simulink model "Correlation_Ex1"  (R2024a)
settings: Solver=VariableStepAuto  StartTime=0.0  StopTime=1024  RelTol=1e-3
InitFcn:
  | F_Length = 16;
  | G_Length = 16;
undefined symbols (not defined in the file): S, vsva2197, xcvc1902
libraries: dspstat3 x1, aieDSP x1, aieUtilities x1, vmcUtilities x1
settings Model: Creator=sdegala  LastModifiedBy=sdegala

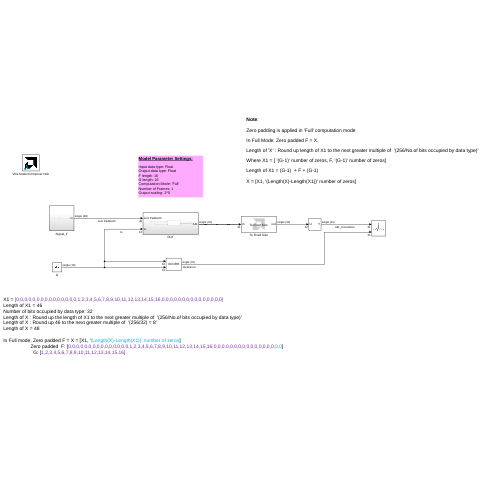
[thumbnail: Simulink's stored preview of the top-level diagram]
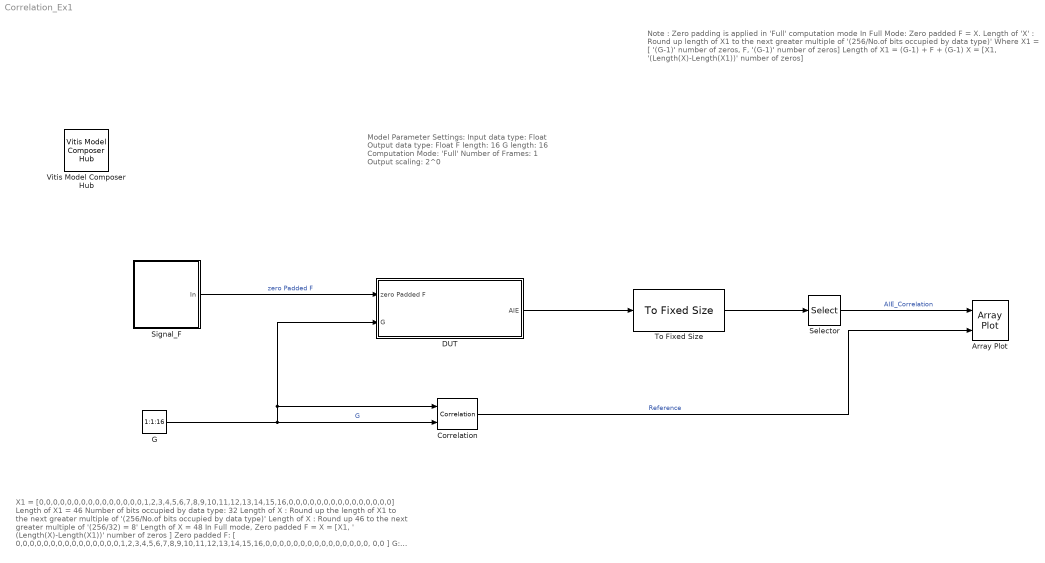
== system Correlation_Ex1 ==
  note: X1 = [0,0,0,0,0,0,0,0,0,0,0,0,0,0,0,1,2,3,4,5,6,7,8,9,10,11,12,13,14,15,16,0,0,0,0,0,0,0,0,0,0,0,0,0,0,0]
      | Length of X1 = 46
      | Number of bits occupied by data type: 32
      | Length of X : Round up the length of X1 to the next greater multiple of '(256/No.of bits occupied by data type)'
      | Length of X : Round up 46 to the next greater multiple of '(256/32) = 8'
      | Length of X = 48
      |
      | In Full mode, Zero padded F = X = [X1, ' (Length(X)-Length(X1))' number of zeros ]
      | Zero padded F: [ 0,0,0,0,0,0,0,0,0,0,0,0,0,0,0,1,2,3,4,5,6,7,8,9,10,11,12,13,14,15,16,0,0,0,0,0,0,0,0,0,0,0,0,0,0,0, 0,0 ]
      | G: [ 1,2,3,4,5,6,7,8,9,10,11,12,13,14,15,16]
  note: Note :
      |
      | Zero padding is applied in 'Full' computation mode
      |
      | In Full Mode: Zero padded F = X.
      |
      | Length of 'X' : Round up length of X1 to the next greater multiple of '(256/No.of bits occupied by data type)'
      |
      | Where X1 = [ '(G-1)' number of zeros, F, '(G-1)' number of zeros]
      |
      | Length of X1 = (G-1) + F + (G-1)
      |
      | X = [X1, '(Length(X)-Length(X1))' number of zeros]
  note: Model Parameter Settings:
      |
      | Input data type: Float
      | Output data type: Float
      | F length: 16
      | G length: 16
      | Computation Mode: 'Full'
      | Number of Frames: 1
      | Output scaling: 2^0
  Array Plot : ArrayPlot  NumInputPorts=2  WindowPosition=[663.000000,396.000000,800.000000,500.000000,]  Visible=on  ScopeFrameLocation=window  YLimits=[-169 1681]  ShowLegend=on
  Correlation : dspstat3/Correlation  domain=Time  roundingMode=Floor  overflowMode=off  outputDataTypeStr=Inherit: Same as accumulator  outputMin=[]  outputMax=[]  outputLastDataTypeStr=Inherit: Same as accumulator
  DUT : Subsystem
  G : Constant  Value=1:1:16  OutDataTypeStr=single  SampleTime=1
  Selector : Selector  InputPortWidth=32  IndexOptions=Index vector (dialog)  Indices=1:1:F_Length+G_Length-1  OutputSizes=1
  Signal_F : Subsystem
  To Fixed Size : aieUtilities/To Fixed Size  Mode=Stop simulation when input variable-size signal is not full  OutputSize=Inherit: Same as input  CopyMethod=Buffer samples to form output  HasStatusOutput=on
  Vitis Model Composer Hub : vmcUtilities/Vitis Model Composer Hub  Tag=genX  CodeGeneration=off  StartColumn=1  NumberOfColumns=1  TargetDirectory=./code  exportDesign=off  analyzeDesign=off  validateDesignOnHw=off  ExportType=AI Engines  IpVendor=xilinx.com  IpLibrary=hls  IpVersion=1.0  IpHWLanguage=Verilog  AieCompilerOptions={}  AieSimulatorOptions={}  CreateTestbench=off  TestbenchStackSize=10  RunRtlSim=off  RunCSim=off  RunAieSim=off  AieSimTimeout=50000  RunAieSimProfiling=off  LaunchVitisAnalyzer=off  PlotOutput=off  RunX86Sim=off  X86SimTimeout=10  GenHwImage=off  GenLibadfXo=off  GenHwValidationCode=off  PlatformType=Not Specified  HwSystemType=Baremetal  HwValidationTarget=hw  ProjDevice=xcvc1902-vsva2197-1LP-e-S  ProjDevicePart=xcvc1902-vsva2197-1LP-e-S  AIEType=AIE  SamplePeriod=-1  ClockFrequency=200  DataPathParallelism=1  xilinxfamily=versalaicore  part=xcvc1902  speed=-1LP-e-S  package=vsva2197  directory=./netlist  testbench=off  incr_netlist=off  synthesis_tool=Vivado  clock_wrapper=Clock Enables  dbl_ovrd=According to Block Masks  dcm_input_clock_period=10  sysclk_period=10  simulink_period=1  eval_field=0  LogFileName=''  NThreads=4
  wires:
  Correlation/1 -> Array Plot/2  "Reference"
  G/1 -> Correlation/2, DUT/2(G), Correlation/1  "G"
  Selector/1 -> Array Plot/1  "AIE_Correlation"
  To Fixed Size/1 -> Selector/1
  Signal_F/1(In) -> DUT/1(zero Padded F)  "zero Padded F"
  DUT/1(AIE) -> To Fixed Size/1

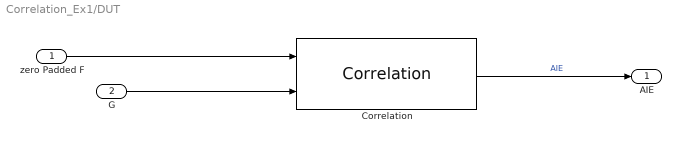
== system Correlation_Ex1/DUT ==
  zero Padded F : Inport
  G : Inport  Port=2
  Correlation : aieDSP/Correlation  AIE_VARIANT=1  data_type_f=float  data_type_g=float  data_type_out=float  compute_mode=Full  f_sample_size=F_Length  g_sample_size=G_Length  num_frames=1  casc_length=1  no_of_kernels=1  shift_coeff=0  rnd_mode=Floor  sat_mode=None  api=0  function_type=0  blockJsonConstraints=[]  blockJsonConstraintsInternal=[]  spec=vmc_corr.json  SerializedMaskParamNames=[]  SerializedMaskParamValues=[]  SerializedMaskParamVisibilities=[]  block_type=Correlation  SerializedMaskParamDataypes=uint|typename|typename|typename|uint|uint|uint|uint|uint|uint|uint|uint|uint|uint|uint  SerializedMaskParamEnumStrArr=0|0|0|0|Full,Same,Valid|0|0|0|0|0|0|Floor,Ceiling,Round to positive infinity,Round to negative infinity,Round symmetrical to infinity,Round symmetrical to zero,Round convergent to even,Round convergent to odd|None,Saturate,Symmetric|0|0  SerializedMaskParamEnumValArr=0|0|0|0|0,1,2|0|0|0|0|0|0|0,1,2,3,4,5,6,7|0,1,3|0|0  SerializedMaskParamVectorArr=0|0|0|0|0|0|0|0|0|0|0|0|0|0|0  SerializedMaskParamKeys=AIE_VARIANT|TT_DATA_F|TT_DATA_G|TT_DATA_OUT|TP_COMPUTE_MODE|TP_F_LEN|TP_G_LEN|TP_NUM_FRAMES|TP_CASC_LEN|TP_PHASES|TP_SHIFT|TP_RND|TP_SAT|TP_API|TP_FUNCT_TYPE
  AIE : Outport
  wires:
  Correlation/1 -> AIE/1  "AIE"
  G/1 -> Correlation/2
  zero Padded F/1 -> Correlation/1

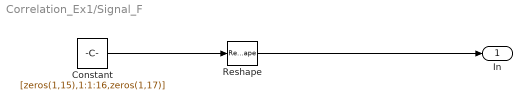
== system Correlation_Ex1/Signal_F ==
  Constant : Constant  Value=[zeros(1,15),1:1:16,zeros(1,17)]  OutDataTypeStr=single  SampleTime=1
  Reshape : Reshape
  In : Outport
  wires:
  Constant/1 -> Reshape/1
  Reshape/1 -> In/1
